simulink model "RadioSYS"  (R2013a)
settings: Solver=ode45  StartTime=0.0  StopTime=1  RelTol=1e-3
libraries: dspsigops x2, commanapbnd3 x1, commrandsrc2 x1
settings Model: Creator=glepenske  LastModifiedBy=glepenske

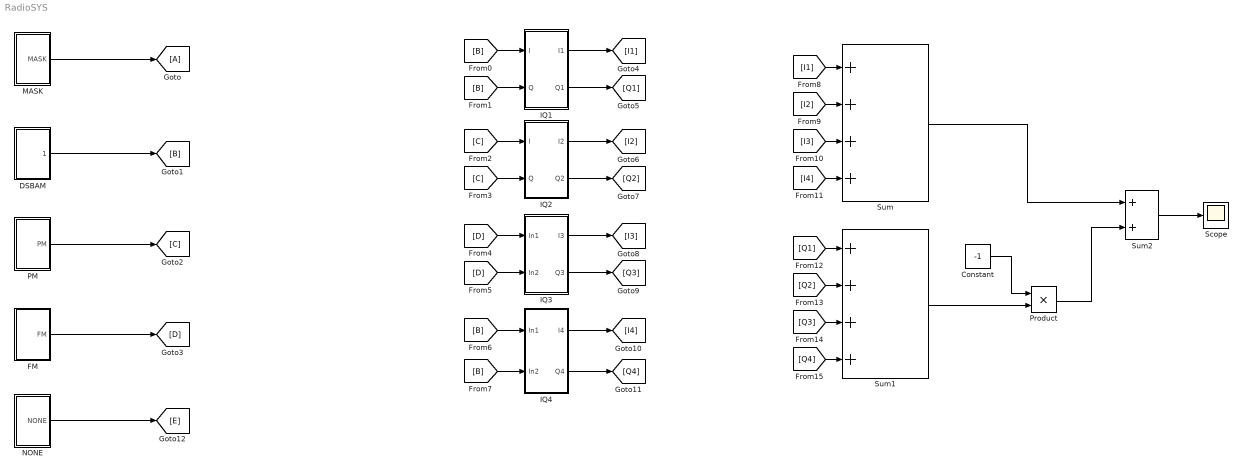
== system RadioSYS ==
  Constant : Constant  Value=-1
  DSBAM : Subsystem
  FM : Subsystem
  IQ1 : Subsystem
  IQ2 : Subsystem
  IQ3 : Subsystem
  IQ4 : Subsystem
  MASK : Subsystem
  NONE : Subsystem
  PM : Subsystem
  Product : Product
  Scope : Scope
      settings: SaveName=ScopeData2
  Sum : Sum  Inputs=++++
  Sum1 : Sum  Inputs=++++
  Sum2 : Sum
  wires:
  MASK/1(MASK) -> [A]
  DSBAM/1("DSBAM ") -> [B]
  FM/1(FM) -> [D]
  [B] -> IQ1/1(I)
  [B] -> IQ1/2(Q)
  [D] -> IQ3/1(In1)
  [D] -> IQ3/2(In2)
  [B] -> IQ4/1(In1)
  [B] -> IQ4/2(In2)
  [C] -> IQ2/1(I)
  [C] -> IQ2/2(Q)
  [I1] -> Sum/1
  Constant/1 -> Product/1
  Sum1/1 -> Product/2
  Sum/1 -> Sum2/1
  Product/1 -> Sum2/2
  [I2] -> Sum/2
  [I3] -> Sum/3
  [I4] -> Sum/4
  [Q1] -> Sum1/1
  [Q2] -> Sum1/2
  [Q3] -> Sum1/3
  [Q4] -> Sum1/4
  Sum2/1 -> Scope/1
  IQ1/1(I1) -> [I1]
  IQ1/2(Q1) -> [Q1]
  IQ2/1(I2) -> [I2]
  IQ2/2(Q2) -> [Q2]
  IQ3/1(I3) -> [I3]
  IQ3/2(Q3) -> [Q3]
  IQ4/1(I4) -> [I4]
  IQ4/2(Q4) -> [Q4]
  PM/1(PM) -> [C]
  NONE/1(NONE) -> [E]

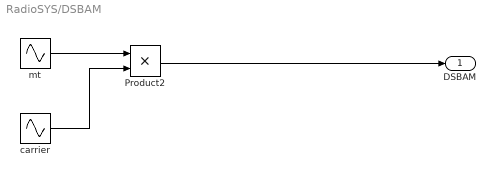
== system RadioSYS/DSBAM ==
  Product2 : Product
  carrier : Sin  Amplitude=0  Frequency=0  Samples=5  SampleTime=0
  mt : Sin  Amplitude=0  Frequency=0  Samples=5  SampleTime=0
  "DSBAM " : Outport
  wires:
  Product2/1 -> "DSBAM "/1
  mt/1 -> Product2/1
  carrier/1 -> Product2/2

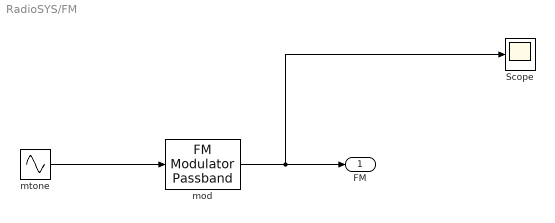
== system RadioSYS/FM ==
  Scope : Scope
      settings: SaveName=ScopeData3  MaxDataPoints=50000000
  mod : commanapbnd3/FM Modulator Passband  Fc=2  Ph=0  Kc=1
  mtone : Sin  Samples=1e5  SampleTime=1e-6
  FM : Outport
  wires:
  mtone/1 -> mod/1
  mod/1 -> Scope/1, FM/1

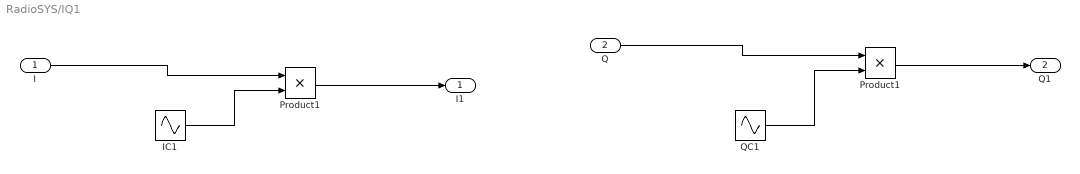
== system RadioSYS/IQ1 ==
  I : Inport
  Q : Inport  Port=2
  "IC1 " : Sin  SineType=Sample based  Frequency=2*pi*10000  Phase=-pi/2  Samples=100  SampleTime=1e-6  Offset=25
  Product1 : Product
  "Product1 " : Product
  QC1 : Sin  SineType=Sample based  Frequency=2*pi*100  Samples=100  SampleTime=1e-6
  I1 : Outport
  Q1 : Outport  Port=2
  wires:
  "Product1 "/1 -> I1/1
  Product1/1 -> Q1/1
  QC1/1 -> Product1/2
  I/1 -> "Product1 "/1
  Q/1 -> Product1/1
  "IC1 "/1 -> "Product1 "/2

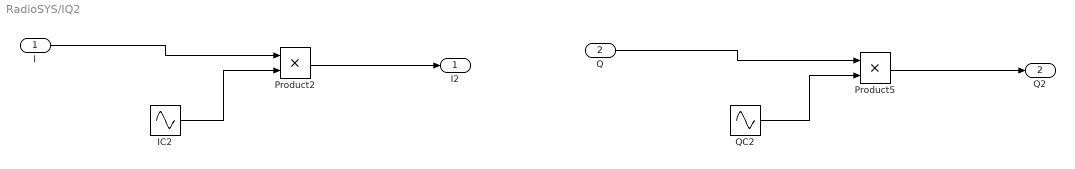
== system RadioSYS/IQ2 ==
  I : Inport
  Q : Inport  Port=2
  IC2 : Sin  Frequency=2*pi*1  Phase=-pi/2  Samples=520  SampleTime=0  Offset=130
  Product2 : Product
  Product5 : Product
  QC2 : Sin  Frequency=2*pi*1  Samples=520  SampleTime=0
  I2 : Outport
  Q2 : Outport  Port=2
  wires:
  Product5/1 -> Q2/1
  QC2/1 -> Product5/2
  Product2/1 -> I2/1
  IC2/1 -> Product2/2
  I/1 -> Product2/1
  Q/1 -> Product5/1

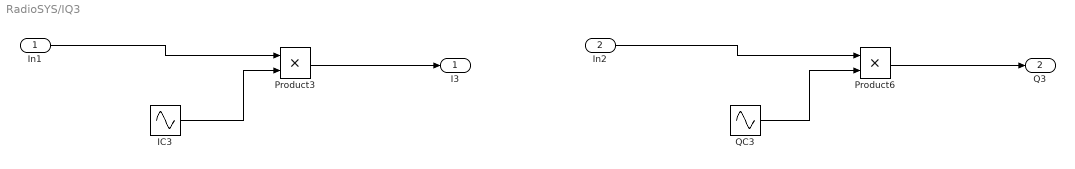
== system RadioSYS/IQ3 ==
  In1 : Inport
  In2 : Inport  Port=2
  IC3 : Sin  Frequency=2*pi*1  Phase=-pi/2  Samples=520  SampleTime=0  Offset=130
  Product3 : Product
  Product6 : Product
  QC3 : Sin  Frequency=2*pi*1  Samples=520  SampleTime=0
  I3 : Outport
  Q3 : Outport  Port=2
  wires:
  IC3/1 -> Product3/2
  Product3/1 -> I3/1
  QC3/1 -> Product6/2
  Product6/1 -> Q3/1
  In2/1 -> Product6/1
  In1/1 -> Product3/1

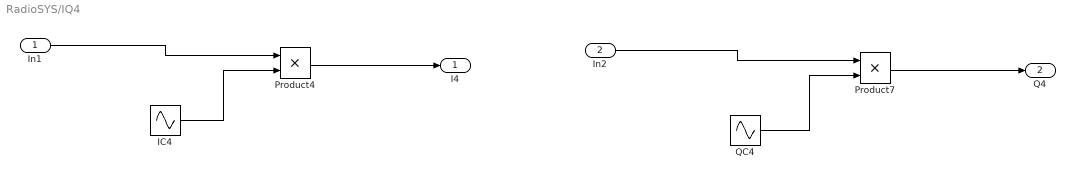
== system RadioSYS/IQ4 ==
  In1 : Inport
  In2 : Inport  Port=2
  IC4 : Sin  Frequency=2*pi*1  Phase=-pi/2  Samples=520  SampleTime=0  Offset=130
  Product4 : Product
  Product7 : Product
  QC4 : Sin  Frequency=2*pi*1  Samples=520  SampleTime=0
  I4 : Outport
  Q4 : Outport  Port=2
  wires:
  Product7/1 -> Q4/1
  QC4/1 -> Product7/2
  Product4/1 -> I4/1
  IC4/1 -> Product4/2
  In1/1 -> Product4/1
  In2/1 -> Product7/1

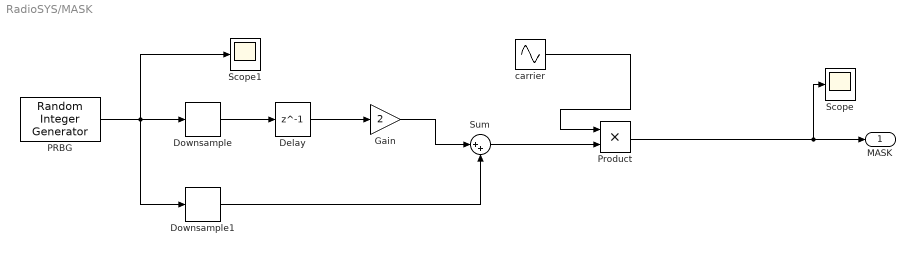
== system RadioSYS/MASK ==
  Delay : Delay  DelayLength=1  InitialCondition=0
  Downsample : dspsigops/Downsample  N=2  phase=0  RateOptions=Enforce single-rate processing  smode=Allow multirate  fmode=Maintain input frame size  ic=0
  Downsample1 : dspsigops/Downsample  N=2  phase=1  RateOptions=Enforce single-rate processing  smode=Allow multirate  fmode=Maintain input frame size  ic=0
  Gain : Gain  Gain=2
  PRBG : commrandsrc2/Random Integer Generator  mul=2  seed=37  Ts=0.001  frameBased=off  sampPerFrame=1  orient=off  outDataType=double
  Product : Product
  Scope : Scope
      settings: MaxDataPoints=5000000
  Scope1 : Scope
  Sum : Sum  Inputs=|++
  carrier : Sin  Amplitude=5  Frequency=6.2832  Phase=0.7854  Samples=10000  SampleTime=0.001
  MASK : Outport
  wires:
  Sum/1 -> Product/2
  Delay/1 -> Gain/1
  Gain/1 -> Sum/1
  PRBG/1 -> Scope1/1, Downsample1/1, Downsample/1
  Downsample/1 -> Delay/1
  carrier/1 -> Product/1
  Product/1 -> Scope/1, MASK/1
  Downsample1/1 -> Sum/2

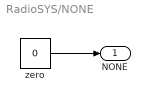
== system RadioSYS/NONE ==
  zero : Constant  Value=0
  NONE : Outport
  wires:
  zero/1 -> NONE/1

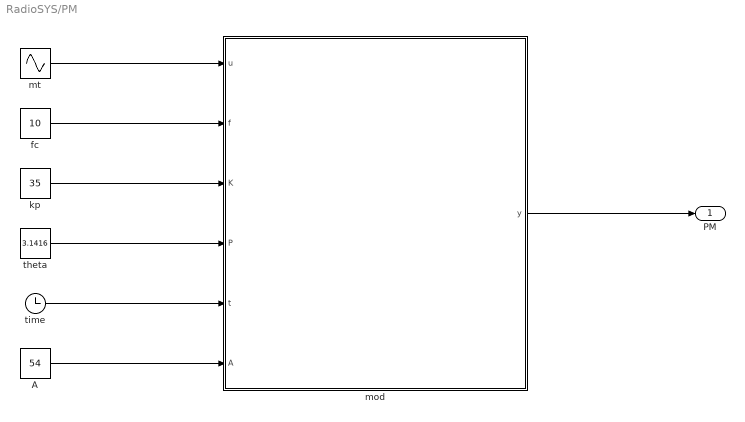
== system RadioSYS/PM ==
  A : Constant  Value=54
  fc : Constant  Value=10
  kp : Constant  Value=35
  mod : MATLAB Function  TreatAsAtomicUnit=on
  mt : Sin  Amplitude=24  Frequency=6.2832  Phase=0.7854  Samples=52e3  SampleTime=1e-05
  theta : Constant  Value=3.1416
  time : Clock
  PM : Outport
  wires:
  mod/1(y) -> PM/1
  theta/1 -> mod/4(P)
  mt/1 -> mod/1(u)
  kp/1 -> mod/3(K)
  fc/1 -> mod/2(f)
  time/1 -> mod/5(t)
  A/1 -> mod/6(A)

== matlab function RadioSYS/PM/mod ==
  data: u input; y output; f input; K input; P input; t input; A input
function y = fcn(u,f,K,P,t,A)
%#codegen

y = A*cos(2*pi*f*t + K*u + P);
